simulink model "I_O_Linear_Model"  (R2012b)
settings: Solver=ode45  StartTime=0.0  StopTime=10.0  RelTol=1e-3
settings Model: Creator=Viktor  LastModifiedBy=Viktor

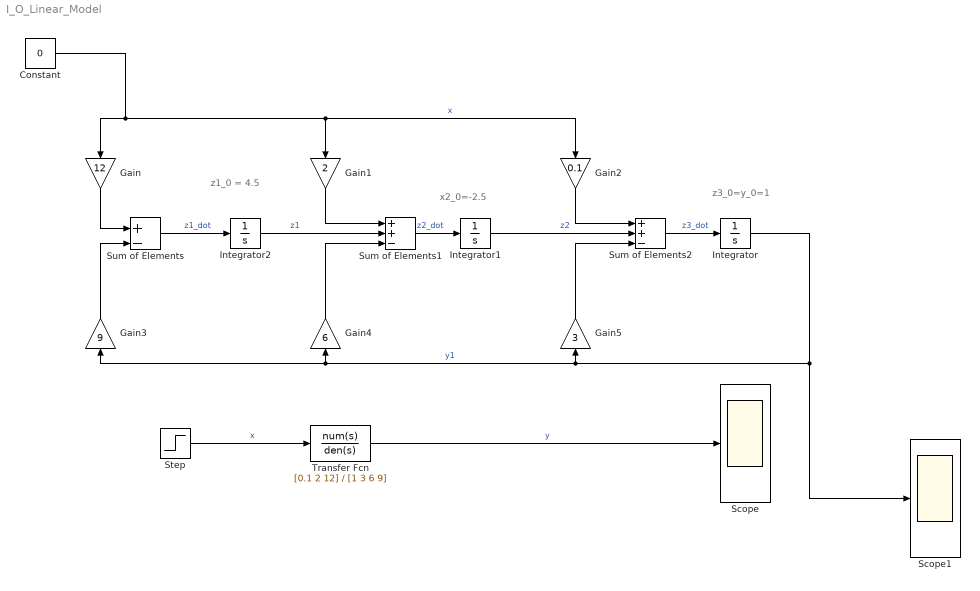
== system I_O_Linear_Model ==
  note: z3_0=y_0=1
  note: x2_0=-2.5
  note: z1_0 = 4.5
  Constant : Constant  Value=0
  Gain : Gain  Gain=12
  Gain1 : Gain  Gain=2
  Gain2 : Gain  Gain=0.1
  Gain3 : Gain  Gain=9
  Gain4 : Gain  Gain=6
  Gain5 : Gain  Gain=3
  Integrator : Integrator  InitialCondition=1
  Integrator1 : Integrator  InitialCondition=2.5
  Integrator2 : Integrator  InitialCondition=4.5
  Scope : Scope
  Scope1 : Scope
  Step : Step  Time=0  SampleTime=0
  Sum of Elements : Sum  Inputs=+|-
  Sum of Elements1 : Sum  Inputs=+|+|-
  Sum of Elements2 : Sum  Inputs=+|+|-
  Transfer Fcn : TransferFcn  Numerator=[0.1 2 12]  Denominator=[1 3 6 9]
  wires:
  Integrator/1 -> Scope1/1, Gain5/1, Gain4/1, Gain3/1  "y1"
  Sum of Elements/1 -> Integrator2/1  "z1_dot"
  Integrator1/1 -> Sum of Elements2/2  "z2"
  Integrator2/1 -> Sum of Elements1/2  "z1"
  Constant/1 -> Gain/1, Gain1/1, Gain2/1  "x"
  Sum of Elements1/1 -> Integrator1/1  "z2_dot"
  Sum of Elements2/1 -> Integrator/1  "z3_dot"
  Gain/1 -> Sum of Elements/1
  Gain3/1 -> Sum of Elements/2
  Gain1/1 -> Sum of Elements1/1
  Gain4/1 -> Sum of Elements1/3
  Gain2/1 -> Sum of Elements2/1
  Gain5/1 -> Sum of Elements2/3
  Step/1 -> Transfer Fcn/1  "x"
  Transfer Fcn/1 -> Scope/1  "y"
